simulink model "MULTILEVEL_13_LEVEL_INVERTER"  (R2025a)
settings: Solver=ode45  StartTime=0.0  StopTime=0.1  RelTol=1e-3  EnableMultiTasking=on
libraries: spsMosfetLib x28, spsDCVoltageSourceLib x7, spsSeriesRLCBranchLib x1, spsVoltageMeasurementLib x1, sps_lib x1
settings Model: Creator=ttt  LastModifiedBy=samar
settings SolverCC: AlgebraicLoopSolver=TrustRegion
settings DataIOCC: LimitDataPoints=on  SaveFormat=Array  SignalLoggingSaveFormat=ModelDataLogs  ReturnWorkspaceOutputs=off
settings OptimizationCC: ExpressionDepthLimit=2147483647.0  LifeSpan=inf
settings DebuggingCC: UnderspecifiedInitializationDetection=Classic  MergeDetectMultiDrivingBlocksExec=none  SolverPrmCheckMsg=warning  FcnCallInpInsideContextMsg=warning  UnconnectedInputMsg=warning  UnconnectedOutputMsg=warning  UnconnectedLineMsg=warning  StateNameClashWarn=warning  SFUnexpectedBacktrackingDiag=warning  SFNoUnconditionalDefaultTransitionDiag=warning  SFExecutionAtInitializationDiag=none  ArithmeticOperatorsInVariantConditions=warning
settings HardwareCC: ProdBitPerPointer=32.0  ProdBitPerSizeT=32.0  ProdBitPerPtrDiffT=32.0  ProdLargestAtomicFloat=None  ProdIntDivRoundTo=Undefined  ProdEndianess=Unspecified  ProdWordSize=32.0  ProdHWDeviceType=32-bit Generic
settings ModelReferenceCC: PropagateSignalLabelsOutOfModel=off
settings SFSimCC: SimUseLocalCustomCode=off  CustomCodeUndefinedFunction=UseInterfaceOnly
settings RTWCC: RTWUseLocalCustomCode=off  GPUComputeCapability=3.5
settings CodeAppCC: StateflowObjectComments=on
settings GRTTargetCC: TargetLangStandard=C89/C90 (ANSI)  CombineOutputUpdateFcns=off  GRTInterface=on
settings ConfigComp: CovMetricSettings=dw  CovSaveCumulativeToWorkspaceVar=on  CovSaveSingleToWorkspaceVar=on  CovExternalEMLEnable=off

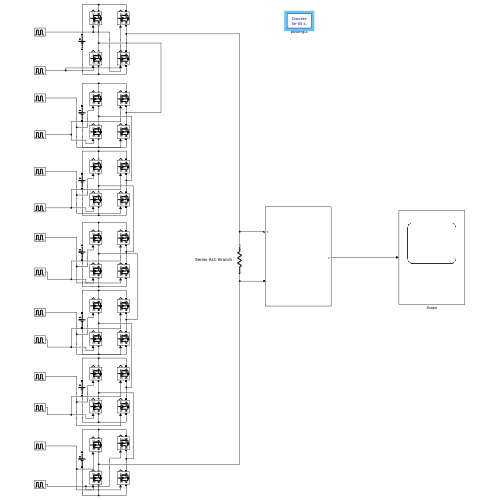
[thumbnail: Simulink's stored preview of the top-level diagram]
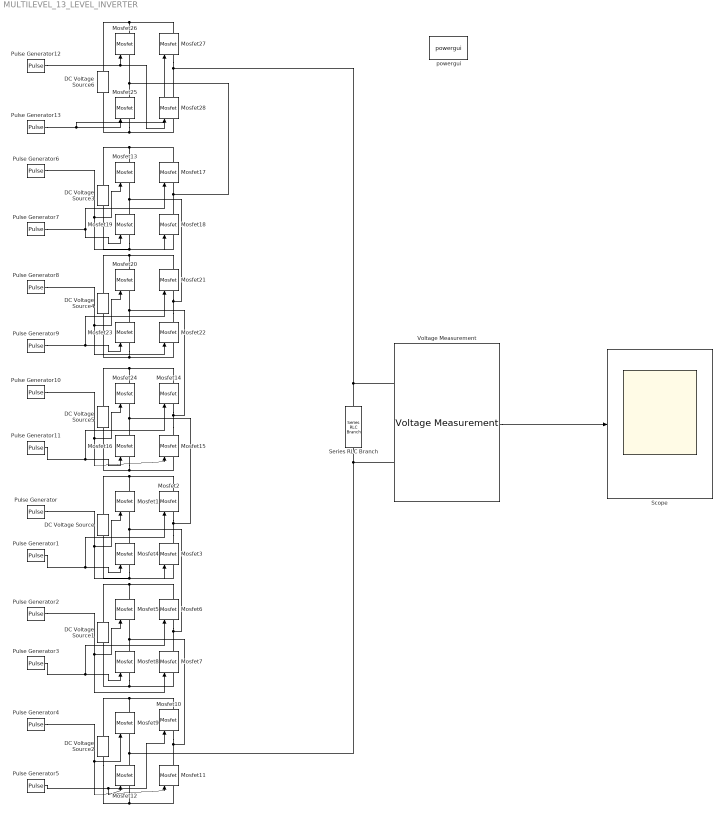
== system MULTILEVEL_13_LEVEL_INVERTER ==
  DC Voltage Source{,1..6} (7 alike) : spsDCVoltageSourceLib/DC Voltage Source  Amplitude=12  Measurements=None
  Mosfet{1..28} (28 alike) : spsMosfetLib/Mosfet  Ron=0.1  Lon=0  Rd=0.01  Vfd=0  IC=0  Rs=1e5  Cs=inf  Measurements=on
  Pulse Generator : DiscretePulseGenerator  PulseType=Time based  Period=1/50  PulseWidth=20  PhaseDelay=0.003
  Pulse Generator1 : DiscretePulseGenerator  PulseType=Time based  Period=1/50  PulseWidth=20  PhaseDelay=0.013
  Pulse Generator10 : DiscretePulseGenerator  PulseType=Time based  Period=1/50  PulseWidth=30  PhaseDelay=0.002
  Pulse Generator11 : DiscretePulseGenerator  PulseType=Time based  Period=1/50  PulseWidth=30  PhaseDelay=0.012
  Pulse Generator12 : DiscretePulseGenerator  PulseType=Time based  Period=1/50  PulseWidth=50
  Pulse Generator13 : DiscretePulseGenerator  PulseType=Time based  Period=1/50  PulseWidth=50
  Pulse Generator2 : DiscretePulseGenerator  PulseType=Time based  Period=1/50  PulseWidth=10  PhaseDelay=0.004
  Pulse Generator3 : DiscretePulseGenerator  PulseType=Time based  Period=1/50  PulseWidth=10  PhaseDelay=0.014
  Pulse Generator4 : DiscretePulseGenerator  PulseType=Time based  Period=1/50  PulseWidth=5  PhaseDelay=0.0045
  Pulse Generator5 : DiscretePulseGenerator  PulseType=Time based  Period=1/50  PulseWidth=5  PhaseDelay=0.0145
  Pulse Generator6 : DiscretePulseGenerator  PulseType=Time based  Period=1/50  PulseWidth=45  PhaseDelay=0.0005
  Pulse Generator7 : DiscretePulseGenerator  PulseType=Time based  Period=1/50  PulseWidth=45  PhaseDelay=0.0105  VectorParams1D=off
  Pulse Generator8 : DiscretePulseGenerator  PulseType=Time based  Period=1/50  PulseWidth=40  PhaseDelay=0.001
  Pulse Generator9 : DiscretePulseGenerator  PulseType=Time based  Period=1/50  PulseWidth=40  PhaseDelay=0.011
  Scope : Scope
      settings: TimeSpan=0.25  ActiveDisplayYMinimum=-4.28568544322529  ActiveDisplayYMaximum=4.2856851497999138
  Series RLC Branch : spsSeriesRLCBranchLib/Series RLC Branch  LConnTagsString=__new0  RConnTagsString=__new0  BranchType=R  Resistance=10000  Inductance=1e-3  SetiL0=off  InitialCurrent=0  Capacitance=1e-6  Setx0=off  InitialVoltage=0  Measurements=None
  Voltage Measurement : spsVoltageMeasurementLib/Voltage Measurement  PhasorSimulation=off  OutputType=Complex  PSBequivalent=0
  powergui : sps_lib/powergui  Priority=1  SimulationMode=Discrete  SampleTime=50e-6  frequency=60  Iterations=50  frequencyindice=0  Pbase=100e6  ErrMax=1e-4  UnitsV=kV  UnitsW=MW  buscounter=0  FunctionMessages=off  echomessages=off  EnableUseOfTLC=off  CurrentSourceSwitches=off  DisableSnubberDevices=off  DisableRonSwitches=off  DisableVfSwitches=off  DisplayEquations=off  AutomaticDiscreteSolvers=off  SolverType=Tustin/Backward Euler (TBE)  Interpol=off  ExternalGateDelay=off  methode=off  Ts=100  x0status=blocks  SPID=off  SwTol=0  HookPort=off  NonlinearTolerance=1e-4  nMaxIteration=100  ContinueOnMaxIteration=off  RestoreLinks=warning  ResistiveCurrentMeasurement=off  Frange=[0:2:500]  Ylog=off  Xlog=on  ShowGrid=off  save=off  variable=ZData  structure=0  ZoomFFT=off  StartTime=0.0  cycles=1  DisplayStyle=1  fundamental=60  FreqAxis=off  MaxFrequency=1000  frequencyindicesteady=1  RmsSteady=1  display=off
  wires:
  Pulse Generator/1 -> Mosfet1/1, Mosfet3/1
  Pulse Generator1/1 -> Mosfet4/1, Mosfet2/1
  Pulse Generator2/1 -> Mosfet7/1, Mosfet5/1
  Pulse Generator3/1 -> Mosfet6/1, Mosfet8/1
  Pulse Generator4/1 -> Mosfet11/1, Mosfet9/1
  Pulse Generator5/1 -> Mosfet12/1, Mosfet10/1
  Voltage Measurement/1 -> Scope/1
  Pulse Generator6/1 -> Mosfet18/1, Mosfet13/1
  Pulse Generator7/1 -> Mosfet19/1, Mosfet17/1
  Pulse Generator8/1 -> Mosfet20/1, Mosfet22/1
  Pulse Generator9/1 -> Mosfet23/1, Mosfet21/1
  Pulse Generator10/1 -> Mosfet15/1, Mosfet24/1
  Pulse Generator11/1 -> Mosfet14/1, Mosfet16/1
  Pulse Generator12/1 -> Mosfet28/1, Mosfet26/1
  Pulse Generator13/1 -> Mosfet25/1, Mosfet27/1
  connections:
  DC Voltage Source/RConn1 -- Mosfet2/RConn1 -- Mosfet1/RConn1
  Mosfet4/LConn1 -- Mosfet3/LConn1 -- DC Voltage Source/LConn1
  Mosfet5/RConn1 -- Mosfet6/RConn1 -- DC Voltage Source1/RConn1
  DC Voltage Source1/LConn1 -- Mosfet7/LConn1 -- Mosfet8/LConn1
  DC Voltage Source2/RConn1 -- Mosfet10/RConn1 -- Mosfet9/RConn1
  Mosfet8/RConn1 -- Mosfet5/LConn1 -- Mosfet11/RConn1 -- Mosfet10/LConn1
  Mosfet4/RConn1 -- Mosfet1/LConn1 -- Mosfet7/RConn1 -- Mosfet6/LConn1
  Mosfet9/LConn1 -- Mosfet12/RConn1 -- Voltage Measurement/LConn2 -- Series RLC Branch/RConn1
  DC Voltage Source3/RConn1 -- Mosfet17/RConn1 -- Mosfet13/RConn1
  Mosfet19/LConn1 -- Mosfet18/LConn1 -- DC Voltage Source3/LConn1
  DC Voltage Source4/RConn1 -- Mosfet21/RConn1 -- Mosfet20/RConn1
  DC Voltage Source4/LConn1 -- Mosfet22/LConn1 -- Mosfet23/LConn1
  DC Voltage Source5/RConn1 -- Mosfet14/RConn1 -- Mosfet24/RConn1
  Mosfet16/LConn1 -- Mosfet15/LConn1 -- DC Voltage Source5/LConn1
  Mosfet15/RConn1 -- Mosfet14/LConn1 -- Mosfet23/RConn1 -- Mosfet20/LConn1
  Mosfet22/RConn1 -- Mosfet21/LConn1 -- Mosfet19/RConn1 -- Mosfet13/LConn1
  Mosfet3/RConn1 -- Mosfet2/LConn1 -- Mosfet16/RConn1 -- Mosfet24/LConn1
  Mosfet12/LConn1 -- DC Voltage Source2/LConn1 -- Mosfet11/LConn1
  Mosfet25/LConn1 -- Mosfet28/LConn1 -- DC Voltage Source6/LConn1
  Mosfet25/RConn1 -- Mosfet18/RConn1 -- Mosfet17/LConn1 -- Mosfet26/LConn1
  Mosfet26/RConn1 -- Mosfet27/RConn1 -- DC Voltage Source6/RConn1
  Mosfet27/LConn1 -- Voltage Measurement/LConn1 -- Series RLC Branch/LConn1 -- Mosfet28/RConn1
